simulink model "FSFB_Int_Sim"  (R2022a)
settings: Solver=VariableStepAuto  StartTime=tspan(1)  StopTime=tspan(2)  RelTol=1e-9
undefined symbols (not defined in the file): r_sim
settings Model: Creator=domin  LastModifiedBy=domin
settings SolverCC: AlgebraicLoopSolver=TrustRegion
settings DebuggingCC: AlgebraicLoopMsg=none  UnconnectedInputMsg=warning  UnconnectedOutputMsg=warning  UnconnectedLineMsg=warning  SFMachineParentedDataDiag=warning
settings RTWCC: DLArmComputeVersion=19.05

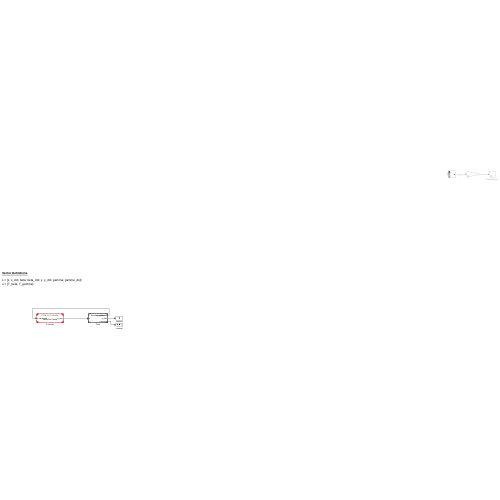
[thumbnail: Simulink's stored preview of the top-level diagram]
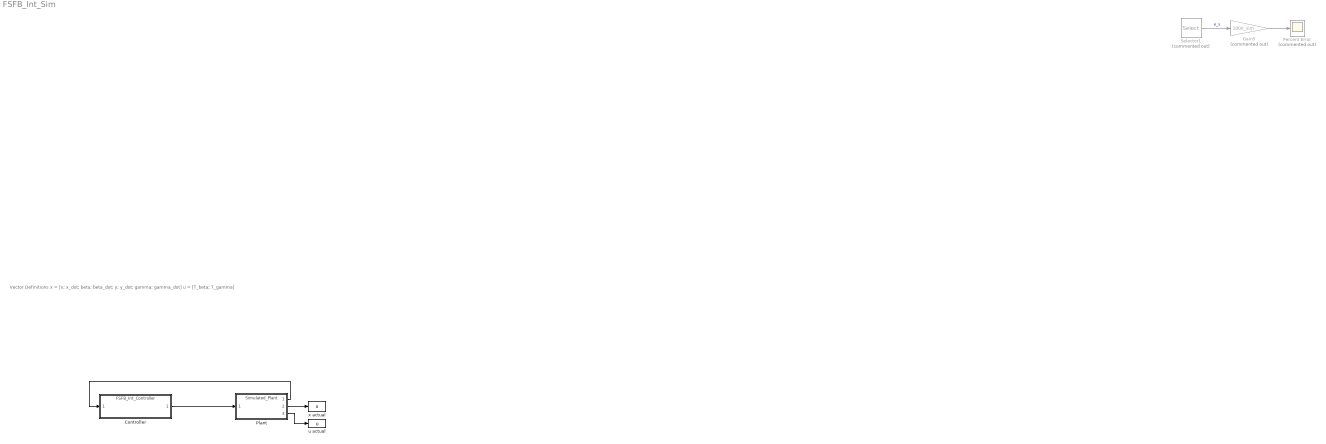
== system FSFB_Int_Sim ==
  note: Vector Definitions
      |
      | x = [x; x_dot; beta; beta_dot; y; y_dot; gamma; gamma_dot]
      | u = [T_beta; T_gamma]
  Controller : ModelReference  ModelNameDialog=FSFB_Int_Controller  SimulationMode=Normal  ModelReferenceVersion=1.2
  Gain5 : Gain  Commented=on  Gain=100/r_sim
  Percent Error : Scope  Commented=on
  Plant : ModelReference  ModelNameDialog=Simulated_Plant  SimulationMode=Normal  ModelReferenceVersion=2.2
  Selector1 : Selector  Commented=on  InputPortWidth=5  IndexOptions=Index vector (dialog)  Indices=[1]  OutputSizes=1
  u actual : ToWorkspace  VariableName=u  SampleTime=-1
  x actual : ToWorkspace  VariableName=x  SampleTime=-1
  wires:
  Gain5/1 -> Percent Error/1
  Selector1/1 -> Gain5/1  "e_x"
  Plant/1 -> Controller/1
  Plant/2 -> x actual/1
  Plant/3 -> u actual/1
  Controller/1 -> Plant/1
